simulink model "Untitled1"  (Simulink 7.9)
settings: Solver=VariableStepDiscrete  StartTime=0.0  StopTime=15000.0  RelTol=1e-3
libraries: simeventslib x1
settings Model: Creator=tsprock3  LastModifiedBy=tsprock3
settings DebuggingCC: SimStateOlderReleaseMsg=warning

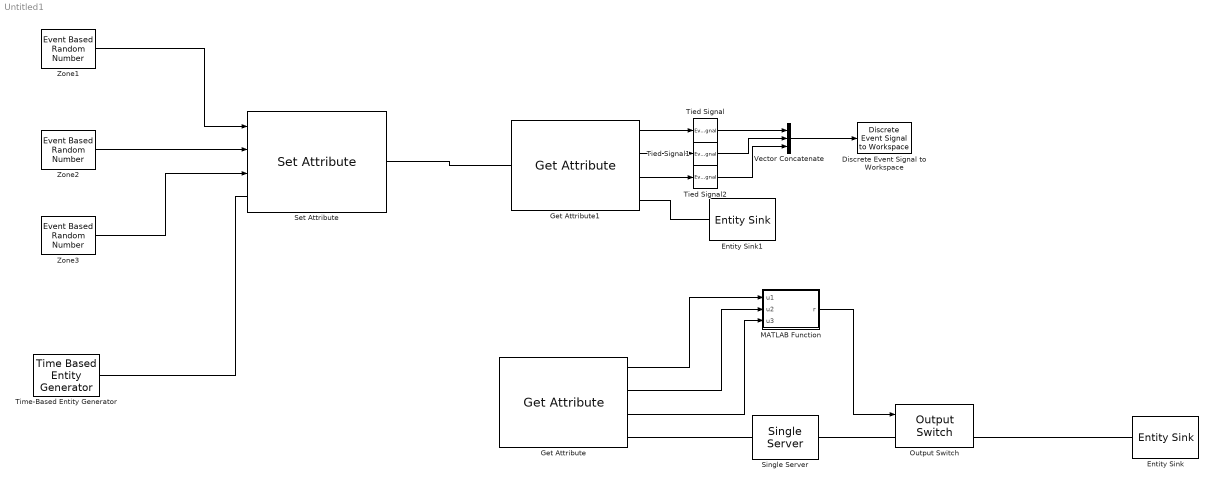
== system Untitled1 ==
  Discrete Event Signal to Workspace : simeventslib/SimEvents Sinks/Discrete Event Signal to Workspace  VariableName=Generated  SaveFormat=Structure With Time  isMonitorOnly=off  isRecordIC=off
  Entity Sink : EntitySink
  Entity Sink1 : EntitySink
  Get Attribute : GetAttribute  AttributeName=Attribute1|Attribute2|Attribute3  AttributeMissing=Error|Error|Error  AttributeDefaultValue=1|1|1  AttributeTreatAsVector=1|1|1  AttributeSendTiming=After entity departure|After entity departure|After entity departure  EvaluatedDefaultAttributeValue={[];[];[]}
      settings: OutputPortMap=o1,o2,o3
  Get Attribute1 : GetAttribute  AttributeName=Attribute1|Attribute2|Attribute3  AttributeMissing=Error|Error|Error  AttributeDefaultValue=1|1|1  AttributeTreatAsVector=1|1|1  AttributeSendTiming=After entity departure|After entity departure|After entity departure  EvaluatedDefaultAttributeValue={[];[];[]}
      settings: OutputPortMap=o1,o2,o3
  MATLAB Function : MATLAB Function  TreatAsAtomicUnit=on
  Output Switch : OutputSwitch  NumberOutputPorts=2  SwitchingCriterion=From signal port p
  Set Attribute : SetAttribute  AttributeName=Attribute1|Attribute2|Attribute3  AttributeFrom=Signal port|Signal port|Signal port  AttributeValue=1|1|1  AttributeTreatAsVector=1|1|1  EvaluatedAttributeValue={[];[];[]}
      settings: InputPortMap=u0,u1,u2
  Single Server : SingleServer  ServiceTime=0
  Tied Signal : EventToTimedSignal
  Tied Signal1 : EventToTimedSignal
  Tied Signal2 : EventToTimedSignal
  Time-Based Entity Generator : TimeBasedEntityGenerator
  Vector Concatenate : Concatenate  NumInputs=3
  Zone1 : EventBasedRandomNumber  Distribution=Triangular  minTri=10  maxTri=97  modeTri=25  scaleGam=8.2957  shapeGam=3.1276  meanNorm=21  stdNorm=16.5  Seed=30384
  Zone2 : EventBasedRandomNumber  Distribution=Triangular  minTri=0  maxTri=186  modeTri=24  meanNorm=58  stdNorm=35.4  Seed=33601
  Zone3 : EventBasedRandomNumber  Distribution=Triangular  minTri=0  maxTri=126  modeTri=18  meanNorm=18  stdNorm=30.8  Seed=36818
  wires:
  Zone1/1 -> Set Attribute/1
  Zone3/1 -> Set Attribute/3
  Zone2/1 -> Set Attribute/2
  Get Attribute/1 -> MATLAB Function/1(u1)
  Get Attribute/2 -> MATLAB Function/2(u2)
  Get Attribute/3 -> MATLAB Function/3(u3)
  MATLAB Function/1(r) -> Output Switch/1
  Vector Concatenate/1 -> Discrete Event Signal to Workspace/1
  Get Attribute1/3 -> Tied Signal2/1
  Get Attribute1/2 -> Tied Signal1/1
  Get Attribute1/1 -> Tied Signal/1
  Tied Signal/1 -> Vector Concatenate/1
  Tied Signal1/1 -> Vector Concatenate/2
  Tied Signal2/1 -> Vector Concatenate/3
  connections:
  Time-Based Entity Generator/RConn1 -- Set Attribute/LConn1
  Get Attribute/RConn1 -- Single Server/LConn1
  Single Server/RConn1 -- Output Switch/LConn1
  Get Attribute1/RConn1 -- Entity Sink1/LConn1
  Output Switch/RConn2 -- Entity Sink/LConn1
  Set Attribute/RConn1 -- Get Attribute1/LConn1

== matlab function MATLAB Function ==
  data: u1 input double; u2 input double; u3 input double; r output double
function r  = fcn(u1, u2, u3)
%#codegen


if (u1+u2+u3 >50) && (u1+u2+u3 < 150)
   r = 1;
else
    r =2;
end
